simulink model "Exemplo_Simulink_Marilia"  (R2023a)
settings: Solver=FixedStepDiscrete  StartTime=0.0  StopTime=10.0  FixedStep=0.1  RelTol=1e-3
InitFcn:
  | warning('off','Simulink:Logging:DatasetRTWGenRootOutputNotSupported');
  | warning('off','Simulink:Logging:DatasetRTWGenStateNotSupported');
StartFcn:
  | warning('off','Simulink:Logging:DatasetRTWGenRootOutputNotSupported');
  | warning('off','Simulink:Logging:DatasetRTWGenStateNotSupported');
StopFcn:
  | warning('on','Simulink:Logging:DatasetRTWGenRootOutputNotSupported');
  | warning('on','Simulink:Logging:DatasetRTWGenStateNotSupported');
CloseFcn:
  | warning('on','Simulink:Logging:DatasetRTWGenRootOutputNotSupported');
  | warning('on','Simulink:Logging:DatasetRTWGenStateNotSupported');
PauseFcn:
  | warning('on','Simulink:Logging:DatasetRTWGenRootOutputNotSupported');
  | warning('on','Simulink:Logging:DatasetRTWGenStateNotSupported');
settings Model: ModifiedByFormat=The MathWorks Inc.  Creator=The MathWorks, Inc.  LastModifiedBy=The MathWorks Inc.
settings SolverCC: AlgebraicLoopSolver=TrustRegion
settings DataIOCC: LimitDataPoints=on  SaveFinalState=on  SaveState=on  SignalLoggingName=logsOut
settings OptimizationCC: DefaultParameterBehavior=Inlined  InlineInvariantSignals=on  ExpressionDepthLimit=2147483647  InitFltsAndDblsToZero=on  LifeSpan=inf
settings DebuggingCC: SaveWithParameterizedLinksMsg=none  CheckExecutionContextPreStartOutputMsg=on  MultiTaskDSMMsg=warning  MultiTaskCondExecSysMsg=none  SigSpecEnsureSampleTimeMsg=none  FcnCallInpInsideContextMsg=warning  UnconnectedInputMsg=warning  UnconnectedOutputMsg=warning  UnconnectedLineMsg=warning  AllowSymbolicDim=off  StateNameClashWarn=warning  StrictBusMsg=ErrorOnBusTreatedAsVector  SFUnexpectedBacktrackingDiag=warning  SFNoUnconditionalDefaultTransitionDiag=warning  SFExecutionAtInitializationDiag=none  ArithmeticOperatorsInVariantConditions=warning
settings HardwareCC: ProdBitPerPointer=32  ProdBitPerSizeT=32  ProdBitPerPtrDiffT=32  ProdLargestAtomicFloat=None  ProdIntDivRoundTo=Undefined  ProdEndianess=Unspecified  ProdWordSize=32  ProdHWDeviceType=32-bit Generic  TargetHWDeviceType=32-bit Generic
settings ModelReferenceCC: UpdateModelReferenceTargets=IfOutOfDate  EnableRefExpFcnMdlSchedulingChecks=on  CheckModelReferenceTargetMessage=none  PropagateSignalLabelsOutOfModel=off
settings SFSimCC: SimUseLocalCustomCode=off  CustomCodeUndefinedFunction=UseInterfaceOnly
settings RTWCC: GenerateReport=on  RTWUseLocalCustomCode=off  LaunchReport=on  DLArmComputeVersion=19.05
settings CodeAppCC: MaxIdLength=100  StateflowObjectComments=on
settings GRTTargetCC: TargetFcnLib=ansi_tfl_tmw.mat  TargetLangStandard=C89/C90 (ANSI)  CombineOutputUpdateFcns=off  GRTInterface=on
settings ConfigComp: CovMetricSettings=dw  CovSaveCumulativeToWorkspaceVar=on  CovSaveSingleToWorkspaceVar=on  CovExternalEMLEnable=off  CovSFcnEnable=off

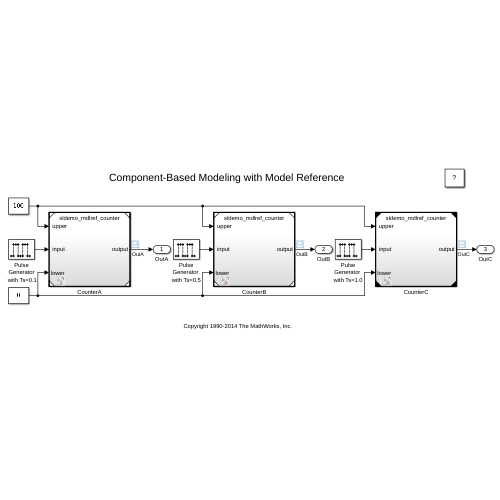
[thumbnail: Simulink's stored preview of the top-level diagram]
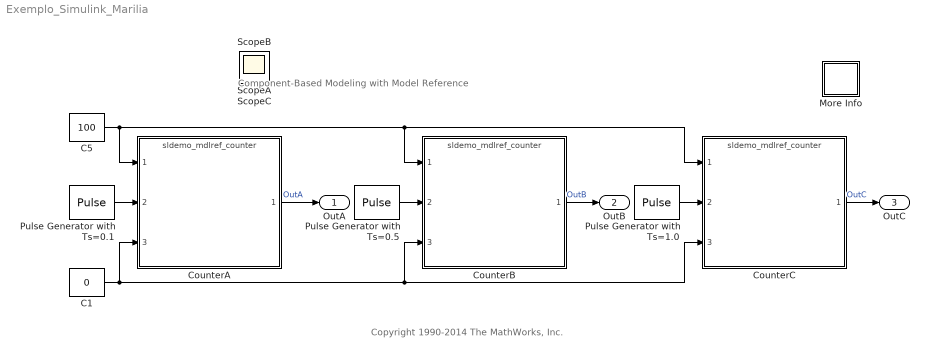
== system Exemplo_Simulink_Marilia ==
  note: Component-Based Modeling with Model Reference
  note: Copyright 1990-2014 The MathWorks, Inc.
  C1 : Constant  Value=0
  C5 : Constant  Value=100
  CounterA : ModelReference  ModelNameDialog=sldemo_mdlref_counter  SimulationMode=Normal  ModelReferenceVersion=6.0
  CounterB : ModelReference  ModelNameDialog=sldemo_mdlref_counter  SimulationMode=Normal  ModelReferenceVersion=6.0
  CounterC : ModelReference  ModelNameDialog=sldemo_mdlref_counter  ModelReferenceVersion=6.0
  More Info : Subsystem
      settings: OpenFcn=showExample('simulink_features/ComponentBasedModelingWithModelReferenceExample')
      mask Display: disp('?')
  Pulse Generator with Ts=0.1 : DiscretePulseGenerator  SampleTime=0.1  VectorParams1D=off
  Pulse Generator with Ts=0.5 : DiscretePulseGenerator  SampleTime=0.5
  Pulse Generator with Ts=1.0 : DiscretePulseGenerator  SampleTime=1.0
  OutA : Outport  VectorParamsAs1DForOutWhenUnconnected=off
  OutB : Outport  Port=2  VectorParamsAs1DForOutWhenUnconnected=off
  OutC : Outport  Port=3  VectorParamsAs1DForOutWhenUnconnected=off
  ScopeA : Scope
  ScopeB : Scope
  ScopeC : Scope
  wires:
  CounterB/1 -> OutB/1  "OutB"
  CounterA/1 -> OutA/1  "OutA"
  CounterC/1 -> OutC/1  "OutC"
  Pulse Generator with Ts=0.1/1 -> CounterA/2
  Pulse Generator with Ts=0.5/1 -> CounterB/2
  Pulse Generator with Ts=1.0/1 -> CounterC/2
  C1/1 -> CounterA/3, CounterB/3, CounterC/3
  C5/1 -> CounterA/1, CounterB/1, CounterC/1

== system Exemplo_Simulink_Marilia/More Info ==
  note: Bus Block Demonstration
  note: This demonstration shows how signals may be grouped and ungrouped while
      | retaining their names.  In this demonstration, 5 signals are created and labelled
      | appropriately.  These signals are then mux'd together to create a bus of signals.
      | This bus of signals is then fed into the Bus Selector block.  Inside of the Bus
      | Selector block, the Pulse and Chirp signals are chosen to be output from the
      | original signal bus.
      |
      | It is possible to place a nest signal buses and then still retrieve the original signal
      | with its label.
